simulink model "testLQR_SteadyRotation"  (R2021a)
settings: Solver=VariableStepAuto  StartTime=0.0  StopTime=Torb  RelTol=1e-3
values from neighbouring files (symbols this model uses):
  Tmax = Fmax*Larm    (= 0.00125)    [control_4.m]
  wz_desired = 20*pi/Torb    [control_4.m]
undefined symbols (not defined in the file or in its folder): K_LQR
libraries: simulink x1, sharedtransform x1
settings Model: DataDictionary=databus.sldd  Creator=Laura  LastModifiedBy=Laura

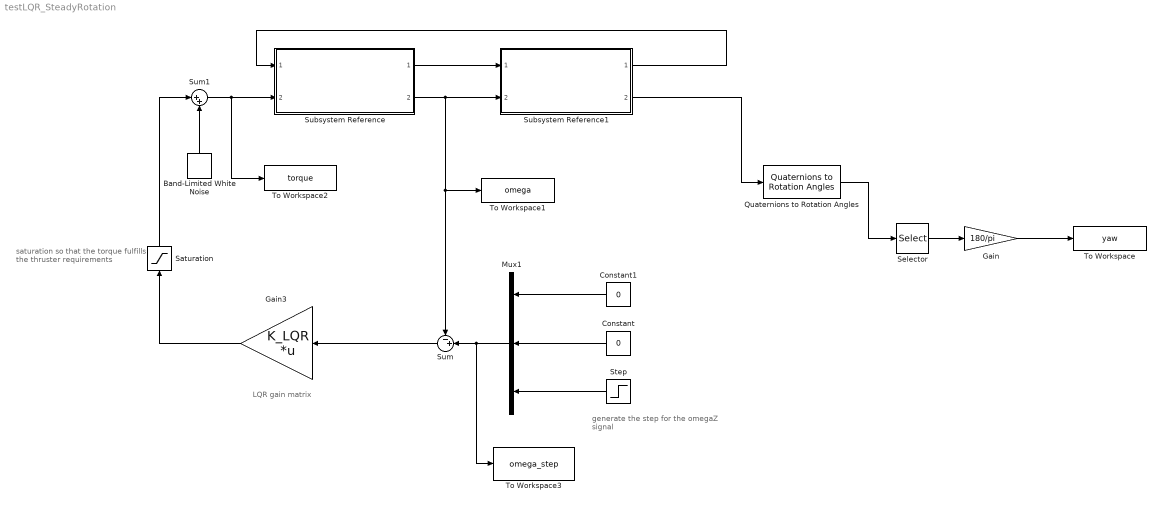
== system testLQR_SteadyRotation ==
  note: saturation so that the torque fulfills the thruster requirements
  note: LQR gain matrix
  note: generate the step
      | for the omegaZ signal
  Band-Limited White Noise : simulink/Sources/Band-Limited White Noise  Cov=[1e-11]  Ts=0.1  seed=[23341]
  Constant : Constant  Value=0
  Constant1 : Constant  Value=0
  Gain : Gain  Gain=180/pi
  Gain3 : Gain  Gain=K_LQR  Multiplication=Matrix(K*u)
  Mux1 : Mux  Inputs=3
  Quaternions to Rotation Angles : sharedtransform/Quaternions to Rotation Angles  rotationOrder=ZYX  aMode=aMode
      settings: SourceProductBaseCode=AE,PW,DR,MT,UV,VE
  Saturation : Saturate  UpperLimit=Tmax  LowerLimit=-Tmax
  Selector : Selector  InputPortWidth=3  IndexOptions=Index vector (dialog)  Indices=[1]  OutputSizes=1
  Step : Step  Time=0  After=wz_desired  SampleTime=0
  Subsystem Reference : Subsystem  ReferencedSubsystem=Dynamics
  Subsystem Reference1 : Subsystem  ReferencedSubsystem=Kinematics
  Sum : Sum  Inputs=-+|
  Sum1 : Sum  Inputs=|++
  To Workspace : ToWorkspace  VariableName=yaw  SaveFormat=Timeseries  SampleTime=-1
  To Workspace1 : ToWorkspace  VariableName=omega  SaveFormat=Timeseries  SampleTime=-1
  To Workspace2 : ToWorkspace  VariableName=torque  SaveFormat=Timeseries  SampleTime=-1
  To Workspace3 : ToWorkspace  VariableName=omega_step  SaveFormat=Timeseries  SampleTime=-1
  wires:
  Sum1/1 -> To Workspace2/1, Subsystem Reference/2
  Subsystem Reference/2 -> Sum/1, To Workspace1/1, Subsystem Reference1/2
  Subsystem Reference1/2 -> Quaternions to Rotation Angles/1
  Gain3/1 -> Saturation/1
  Sum/1 -> Gain3/1
  Subsystem Reference/1 -> Subsystem Reference1/1
  Selector/1 -> Gain/1
  Subsystem Reference1/1 -> Subsystem Reference/1
  Band-Limited White Noise/1 -> Sum1/2
  Step/1 -> Mux1/3
  Constant/1 -> Mux1/2
  Constant1/1 -> Mux1/1
  Mux1/1 -> To Workspace3/1, Sum/2
  Saturation/1 -> Sum1/1
  Quaternions to Rotation Angles/1 -> Selector/1
  Gain/1 -> To Workspace/1
